simulink model "Stanley_model"  (R2012b)
settings: Solver=ode3  StartTime=0.0  StopTime=8  FixedStep=0.05  RelTol=1e-3
values from neighbouring files (symbols this model uses):
  init_angle = pi/2    (= 1.57079632679)    [Stanley.m]
  start_index = i_min(1)    [Stanley.m]
settings Model: Creator=Duytan2804  LastModifiedBy=Duytan2804

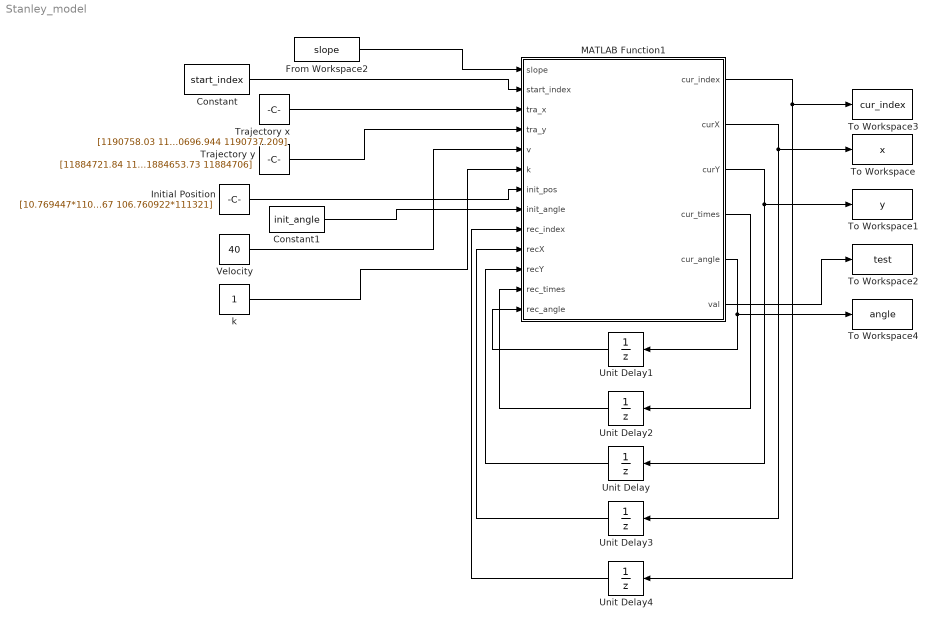
== system Stanley_model ==
  Constant : Constant  Value=start_index
  Constant1 : Constant  Value=init_angle
  From Workspace2 : FromWorkspace  VariableName=slope  SampleTime=0
  Initial Position : Constant  Value=[10.769447*110567 106.760922*111321]
  MATLAB Function1 : MATLAB Function  TreatAsAtomicUnit=on
  To Workspace : ToWorkspace  VariableName=x  SampleTime=-1
  To Workspace1 : ToWorkspace  VariableName=y  SampleTime=-1
  To Workspace2 : ToWorkspace  VariableName=test  SampleTime=-1
  To Workspace3 : ToWorkspace  VariableName=cur_index  SampleTime=-1
  To Workspace4 : ToWorkspace  VariableName=angle  SampleTime=-1
  Trajectory x : Constant  Value=[1190758.03 1190768.408 1190783.537 1190801.523 1190754.863 1190716.183 1190696.944 1190737.209]
  Trajectory y : Constant  Value=[11884721.84 11884710.52 11884701.22 11884678.87 11884656.58 11884632.74 11884653.73 11884706]
  Unit Delay{,1..4} (5 alike) : UnitDelay  SampleTime=-1
  Velocity : Constant  Value=40
  k : Constant
  wires:
  Initial Position/1 -> MATLAB Function1/7(init_pos)
  Velocity/1 -> MATLAB Function1/5(v)
  k/1 -> MATLAB Function1/6(k)
  MATLAB Function1/5(cur_angle) -> To Workspace4/1, Unit Delay1/1
  Unit Delay1/1 -> MATLAB Function1/13(rec_angle)
  MATLAB Function1/4(cur_times) -> Unit Delay2/1
  Unit Delay2/1 -> MATLAB Function1/12(rec_times)
  MATLAB Function1/3(curY) -> Unit Delay/1, To Workspace1/1
  Unit Delay/1 -> MATLAB Function1/11(recY)
  MATLAB Function1/2(curX) -> Unit Delay3/1, To Workspace/1
  Unit Delay3/1 -> MATLAB Function1/10(recX)
  MATLAB Function1/1(cur_index) -> Unit Delay4/1, To Workspace3/1
  Unit Delay4/1 -> MATLAB Function1/9(rec_index)
  From Workspace2/1 -> MATLAB Function1/1(slope)
  Constant/1 -> MATLAB Function1/2(start_index)
  Constant1/1 -> MATLAB Function1/8(init_angle)
  MATLAB Function1/6(val) -> To Workspace2/1
  Trajectory x/1 -> MATLAB Function1/3(tra_x)
  Trajectory y/1 -> MATLAB Function1/4(tra_y)

== matlab function Stanley_model/MATLAB Function1 ==
  data: cur_index output; curX output; curY output; slope input; cur_times output; start_index input; tra_x input; tra_y input; v input; k input; init_pos input; init_angle input; rec_index input; recX input; recY input; rec_times input; rec_angle input; cur_angle output; val output
function [cur_index, curX, curY, cur_times, cur_angle, val] = Stanley(slope, start_index, tra_x, tra_y, v, k, init_pos, init_angle, rec_index, recX, recY, rec_times, rec_angle)
if (rec_index > (length(tra_x) - 1))
    cur_index = rec_index; 
    cur_angle = rec_angle;
    curX = recX + v*cos(cur_angle)*0.05;
    curY = recY + v*sin(cur_angle)*0.05;
    cur_times = rec_times + 1;
    line = 0; val = 0;
else
    if (rec_times == 0)
        recX = init_pos(1); recY = init_pos(2);
        rec_index = start_index;
        rec_angle = init_angle;
    end
    
    perpen_vct1 = tra_x(rec_index + 1) - tra_x(rec_index); 
    perpen_vct2 = tra_y(rec_index + 1) - tra_y(rec_index);
    vct_d1 = tra_x(rec_index) - recX; 
    vct_d2 = tra_y(rec_index) - recY;
    
    if ((-perpen_vct1) ~= 0)
        line = (- perpen_vct1)*(perpen_vct2*recX - perpen_vct1*recY - (perpen_vct2*tra_x(rec_index) - perpen_vct1*tra_y(rec_index)));
    else
        line = (perpen_vct2)*(perpen_vct2*recX  - (perpen_vct2*tra_x(rec_index) - perpen_vct1*tra_y(rec_index)));
    end
    
    x = abs(perpen_vct2*vct_d1 - perpen_vct1*vct_d2)/sqrt(perpen_vct1^2 + perpen_vct2^2);
    
    phi = -rec_angle + slope(rec_index);
    %cur_angle = phi + atan(k*x/v) + rec_angle;
    if ((slope(rec_index) <= -pi/2) || (slope(rec_index) >= pi/2))
        cur_angle = phi + sign(line)*atan(k*x/v) + rec_angle;
    else
        cur_angle = phi - sign(line)*atan(k*x/v) + rec_angle;
    end
    val = x;
%     if ((cur_angle - rec_angle) > pi/3)
%         cur_angle = rec_angle + pi/3;
%     end
%     if ((cur_angle - rec_angle) < -pi/3)
%         cur_angle = rec_angle - pi/3;
%     end
    curX = recX + v*cos(cur_angle)*0.05;
    curY = recY + v*sin(cur_angle)*0.05;
    if (rec_times ~= 0)
        d = [0 0]; 
        d(1) = sqrt((recX-tra_x(rec_index))^2 + (recY-tra_y(rec_index))^2);
        d(2) = sqrt((recX-tra_x(rec_index+1))^2 + (recY-tra_y(rec_index+1))^2);
         % Khoang cach duoc tinh tu diem xuat phat den tat ca cac diem trong quy dao
        if (d(2)/d(1) < 1/3)
            rec_index = rec_index + 1;
        end
    end
    cur_index = rec_index;
    cur_times = rec_times + 1;
    
end
